simulink model "AsteroidImpact_2018a_original"  (R2019a)
settings: Solver=ode4  StartTime=0.0  StopTime=45  FixedStep=0.001  RelTol=1e-3
undefined symbols (not defined in the file or in its folder): g_, K, m_
libraries: eeGeneralControl x2
settings Model: Creator=KNMALE002  LastModifiedBy=Jamie Aronson
settings DataIOCC: SaveOutput=off  SignalLogging=off  DSMLogging=off  ReturnWorkspaceOutputs=off  TimeSaveName=simulation_time
settings DebuggingCC: ArithmeticOperatorsInVariantConditions=warning

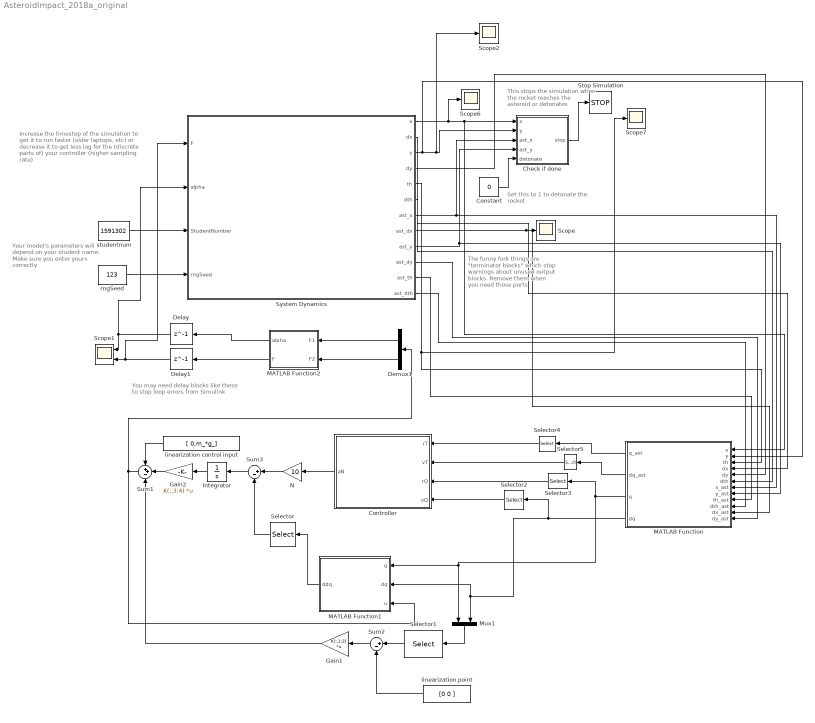
== system AsteroidImpact_2018a_original ==
  note: Increase the timestep of the simulation to get it to run faster (older laptops, etc) or decrease it to get less lag for the (discrete parts of) your controller (higher sampling rate)
  note: You may need delay blocks like these to stop loop errors from Simulink
  note: Your model's parameters will depend on your student name. Make sure you enter yours correctly
  note: The funny fork things are "terminator blocks" which stop warnings about unused output blocks. Remove them when you need those ports
  note: This stops the simulation when the rocket reaches the asteroid or detonates
  note: Set this to 1 to detonate the rocket
  Check if done : MATLAB Function  TreatAsAtomicUnit=on
  Constant : Constant  Value=0
  Controller : MATLAB Function  TreatAsAtomicUnit=on
  Delay : Delay  DelayLength=1  InitialCondition=0
  Delay1 : Delay  DelayLength=1  InitialCondition=10000
  Demux1 : Demux  Outputs=2
  Gain1 : Gain  Gain=K(:,1:2)  Multiplication=Matrix(K*u)
  Gain2 : Gain  Gain=K(:,3:4)  Multiplication=Matrix(K*u)
  Integrator : Integrator
  MATLAB Function : MATLAB Function  TreatAsAtomicUnit=on
  MATLAB Function1 : MATLAB Function  TreatAsAtomicUnit=on
  MATLAB Function2 : MATLAB Function  TreatAsAtomicUnit=on
  Mux1 : Mux  Inputs=2
  N : Gain  Gain=10
  Scope{,2,6..7} (4 alike) : Scope
  Scope1 : Scope  NumInputPorts=2
  Selector{,2..5} (5 alike) : Selector  InputPortWidth=3  IndexOptions=Index vector (dialog)  Indices=[1 2]  OutputSizes=1
  Selector1 : Selector  InputPortWidth=6  IndexOptions=Index vector (dialog)  Indices=[3 6]  OutputSizes=1
  Stop Simulation : Stop
  Sum1 : Sum  Inputs=++-
  Sum2 : Sum  Inputs=|+-
  Sum3 : Sum  Inputs=|+-
  System Dynamics : Subsystem  TreatAsAtomicUnit=on  mask{Value=1}
      mask prompts: Value "Enter mode (1, 2 or 3)"
      mask TypeOptions Value: ScenarioVar/Value
      mask Display: image('lander.jpg');
  linearization control input : Constant  Value=[ 0,m_*g_]
  linearization point : Constant  Value=[0 0 ]
  rngSeed : Constant  Value=123
  studentnum : Constant  Value=1591302
  wires:
  studentnum/1 -> System Dynamics/3(StudentNumber)
  System Dynamics/1(x) -> Scope6/1, MATLAB Function/1(x), Check if done/1(x)
  rngSeed/1 -> System Dynamics/4(rngSeed)
  System Dynamics/3(y) -> MATLAB Function/2(y), Scope2/1, Check if done/2(y)
  System Dynamics/12(ast_dth) -> MATLAB Function/10(dth_ast)
  System Dynamics/7(ast_x) -> MATLAB Function/7(x_ast), Check if done/3(ast_x)
  System Dynamics/9(ast_y) -> MATLAB Function/8(y_ast), Check if done/4(ast_y)
  System Dynamics/8(ast_dx) -> MATLAB Function/11(dx_ast), Scope/1
  System Dynamics/11(ast_th) -> MATLAB Function/9(th_ast)
  Constant/1 -> Check if done/5(detonate)
  System Dynamics/4(dy) -> MATLAB Function/5(dy)
  System Dynamics/10(ast_dy) -> MATLAB Function/12(dy_ast)
  System Dynamics/2(dx) -> MATLAB Function/4(dx)
  System Dynamics/6(dth) -> MATLAB Function/6(dth)
  MATLAB Function/1(q_ast) -> Selector4/1
  MATLAB Function/2(dq_ast) -> Selector5/1
  MATLAB Function/3(q) -> Mux1/1, MATLAB Function1/1(q), Selector3/1
  MATLAB Function/4(dq) -> MATLAB Function1/2(dq), Mux1/2, Selector2/1
  Controller/1(aN) -> N/1
  N/1 -> Sum3/1
  linearization control input/1 -> Sum1/1
  Gain2/1 -> Sum1/2
  Mux1/1 -> Selector1/1
  linearization point/1 -> Sum2/2
  Sum2/1 -> Gain1/1
  Gain1/1 -> Sum1/3
  Selector1/1 -> Sum2/1
  Sum1/1 -> MATLAB Function1/3(u), Demux1/1
  MATLAB Function1/1(ddq) -> Selector/1
  Selector/1 -> Sum3/2
  System Dynamics/5(th) -> Scope7/1, MATLAB Function/3(th)
  Selector2/1 -> Controller/4(vQ)
  Selector3/1 -> Controller/3(rQ)
  Selector4/1 -> Controller/1(rT)
  Selector5/1 -> Controller/2(vT)
  Demux1/1 -> MATLAB Function2/1(F1)
  Demux1/2 -> MATLAB Function2/2(F2)
  MATLAB Function2/2(F) -> Delay1/1
  Delay/1 -> System Dynamics/2(alpha), Scope1/1
  Integrator/1 -> Gain2/1
  Sum3/1 -> Integrator/1
  MATLAB Function2/1(alpha) -> Delay/1
  Delay1/1 -> System Dynamics/1(F), Scope1/2
  Check if done/1(stop) -> Stop Simulation/1

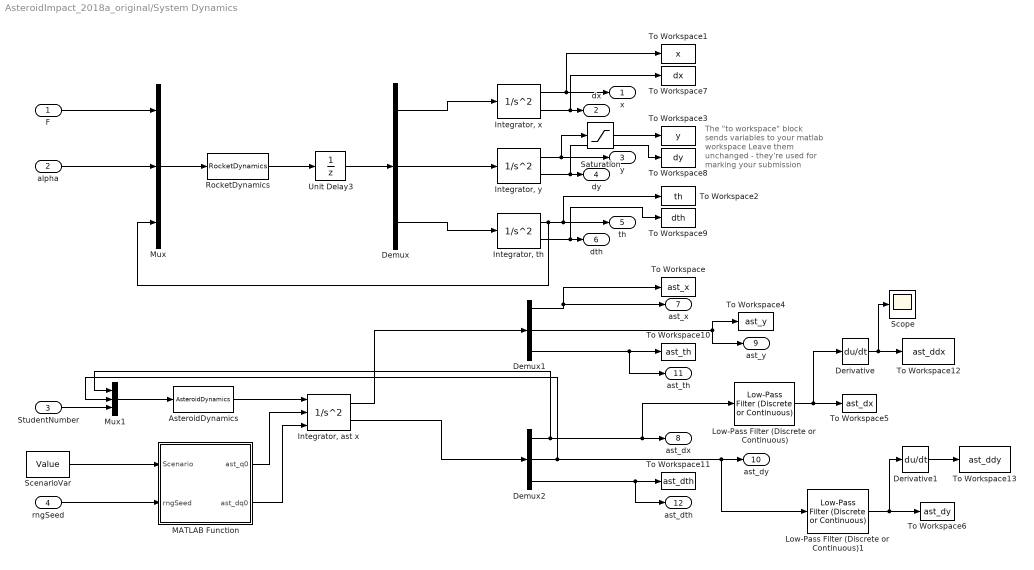
== system AsteroidImpact_2018a_original/System Dynamics ==
  note: The "to workspace" block sends variables to your matlab workspace
      |
      | Leave them unchanged - they're used for marking your submission
  F : Inport
  alpha : Inport  Port=2
  StudentNumber : Inport  Port=3
  rngSeed : Inport  Port=4
  AsteroidDynamics : MATLABFcn  MATLABFcn=AsteroidDynamics  OutputDimensions=3
  Demux : Demux  Outputs=3
  Demux1 : Demux  Outputs=3
  Demux2 : Demux  Outputs=3
  Derivative : Derivative
  Derivative1 : Derivative
  "Integrator, th" : SecondOrderIntegrator  ICX=0  ICDXDT=0
  "Integrator, x" : SecondOrderIntegrator  ICX=0
  "Integrator, y" : SecondOrderIntegrator  ICX=0
  "Integrator, ast x" : SecondOrderIntegrator  ICSourceX=external  ICX=x0  ICSourceDXDT=external
  Low-Pass Filter (Discrete or Continuous) : eeGeneralControl/Low-Pass Filter (Discrete or Continuous)  K=1  T=1  B=inf  A=-inf  Ts=0
      settings: SourceProductName=Simscape Electrical
  Low-Pass Filter (Discrete or Continuous)1 : eeGeneralControl/Low-Pass Filter (Discrete or Continuous)  K=1  T=1  B=inf  A=-inf  Ts=0
      settings: SourceProductName=Simscape Electrical
  MATLAB Function : MATLAB Function  TreatAsAtomicUnit=on
  Mux : Mux  Inputs=3
  Mux1 : Mux  Inputs=3
  RocketDynamics : MATLABFcn  MATLABFcn=RocketDynamics  Output1D=off
  Saturation : Saturate  UpperLimit=10000  LowerLimit=0
  ScenarioVar : Constant  Value=Value
  Scope : Scope
  To Workspace : ToWorkspace  VariableName=ast_x  SampleTime=-1
  To Workspace1 : ToWorkspace  VariableName=x  SampleTime=-1
  To Workspace10 : ToWorkspace  VariableName=ast_th  SampleTime=-1
  To Workspace11 : ToWorkspace  VariableName=ast_dth  SampleTime=-1
  To Workspace12 : ToWorkspace  VariableName=ast_ddx  SaveFormat=Timeseries  SampleTime=-1
  To Workspace13 : ToWorkspace  VariableName=ast_ddy  SaveFormat=Timeseries  SampleTime=-1
  To Workspace2 : ToWorkspace  VariableName=th  SampleTime=-1
  To Workspace3 : ToWorkspace  VariableName=y  SampleTime=-1
  To Workspace4 : ToWorkspace  VariableName=ast_y  SampleTime=-1
  To Workspace5 : ToWorkspace  VariableName=ast_dx  SampleTime=-1
  To Workspace6 : ToWorkspace  VariableName=ast_dy  SampleTime=-1
  To Workspace7 : ToWorkspace  VariableName=dx  SampleTime=-1
  To Workspace8 : ToWorkspace  VariableName=dy  SampleTime=-1
  To Workspace9 : ToWorkspace  VariableName=dth  SampleTime=-1
  Unit Delay3 : UnitDelay  SampleTime=-1  HasFrameUpgradeWarning=on
  x : Outport  PortDimensions=1
  dx : Outport  Port=2  PortDimensions=1
  y : Outport  Port=3  PortDimensions=1
  dy : Outport  Port=4  PortDimensions=1
  th : Outport  Port=5  PortDimensions=1
  dth : Outport  Port=6  PortDimensions=1
  ast_x : Outport  Port=7  PortDimensions=1
  ast_dx : Outport  Port=8  PortDimensions=1
  ast_y : Outport  Port=9  PortDimensions=1
  ast_dy : Outport  Port=10  PortDimensions=1
  ast_th : Outport  Port=11  PortDimensions=1
  ast_dth : Outport  Port=12  PortDimensions=1
  wires:
  "Integrator, th"/1 -> th/1, To Workspace2/1, Mux/3
  Demux/1 -> "Integrator, x"/1
  Demux/2 -> "Integrator, y"/1
  Demux/3 -> "Integrator, th"/1
  "Integrator, x"/1 -> x/1, To Workspace1/1
  "Integrator, x"/2 -> To Workspace7/1, dx/1
  "Integrator, y"/2 -> To Workspace8/1, dy/1
  "Integrator, th"/2 -> To Workspace9/1, dth/1
  Mux/1 -> RocketDynamics/1
  RocketDynamics/1 -> Unit Delay3/1
  rngSeed/1 -> MATLAB Function/2(rngSeed)
  ScenarioVar/1 -> MATLAB Function/1(Scenario)
  F/1 -> Mux/1
  alpha/1 -> Mux/2
  Demux1/3 -> To Workspace10/1, ast_th/1
  Demux2/3 -> ast_dth/1, To Workspace11/1
  Mux1/1 -> AsteroidDynamics/1
  AsteroidDynamics/1 -> "Integrator, ast x"/1
  "Integrator, ast x"/1 -> Demux1/1
  "Integrator, ast x"/2 -> Demux2/1
  Demux1/1 -> To Workspace/1, ast_x/1
  Demux2/1 -> Mux1/1, Low-Pass Filter (Discrete or Continuous)/1, ast_dx/1
  Demux2/2 -> Mux1/2, Low-Pass Filter (Discrete or Continuous)1/1, ast_dy/1
  MATLAB Function/1(ast_q0) -> "Integrator, ast x"/2
  MATLAB Function/2(ast_dq0) -> "Integrator, ast x"/3
  StudentNumber/1 -> Mux1/3
  Unit Delay3/1 -> Demux/1
  "Integrator, y"/1 -> y/1, Saturation/1
  Demux1/2 -> To Workspace4/1, ast_y/1
  Saturation/1 -> To Workspace3/1
  Low-Pass Filter (Discrete or Continuous)/1 -> Derivative/1, To Workspace5/1
  Derivative/1 -> Scope/1, To Workspace12/1
  Low-Pass Filter (Discrete or Continuous)1/1 -> Derivative1/1, To Workspace6/1
  Derivative1/1 -> To Workspace13/1

== matlab function AsteroidImpact_2018a_original/System Dynamics/MATLAB Function ==
  data: ast_q0 output; ast_dq0 output; Scenario input; rngSeed input
function [ast_q0, ast_dq0] = fcn(Scenario, rngSeed)
rng(rngSeed);
if (Scenario == 1)
    x0 = -3000;
    y0 =  5000;
    th0 =   0;
    dx0 = 182;
    dy0 = 0;
    dth0 = 0;

elseif (Scenario == 2)
    x0 = -2000 + rand_within_plus_minus(100);
    y0 = 4000 + rand_within_plus_minus(100); 
    th0 = 0;
    dx0 = 170;
    dy0 = 0;
    dth0 = 0.1;


elseif (Scenario == 3)
    x0 = -2500;
    y0 = 3000;
    th0 = 0;
    dx0 = 160;
    dy0 = 100;
    dth0 = deg2rad(rand_within_plus_minus(20)); % rad/sec

else
    error('You entered an invalid mode -- make sure Scenario = 1, 2 or 3')
end

ast_q0  = [ x0;  y0;  th0];
ast_dq0 = [dx0; dy0; dth0];

end

% calling rand_within_plus_minus(100) returns a number between -100 and 100
function n = rand_within_plus_minus(interval)
    n = (rand - 0.5) * 2 * interval;
end

== matlab function AsteroidImpact_2018a_original/Controller ==
  data: aN output; rT input; vT input; rQ input; vQ input
function aN = pNav(rT, vT, rQ, vQ)
% this produces an acceleration which the controller should track
R = rT - rQ;
Rtemp = [R; 0];
Vr = vT - vQ;
Vtemp = [Vr; 0];
omega = cross(Rtemp, Vtemp) / dot(Rtemp, Rtemp);
temp = cross(Vtemp, omega);
aN = temp(1:2);

== matlab function AsteroidImpact_2018a_original/MATLAB Function ==
  data: x input; q_ast output; y input; th input; dx input; dy input; dth input; x_ast input; y_ast input; th_ast input; dth_ast input; dx_ast input; dy_ast input; dq_ast output; q output; dq output
function [q_ast, dq_ast, q, dq] = fcn(x,y,th,dx,dy,dth,x_ast, y_ast,th_ast,dth_ast, dx_ast, dy_ast)

q_ast = [x_ast; y_ast;th_ast];
dq_ast = [dx_ast; dy_ast;dth_ast]
q = [x;y;th];
dq = [dx;dy;dth];

== matlab function AsteroidImpact_2018a_original/Check if done ==
  data: x input; stop output; y input; ast_x input; ast_y input; detonate input
function stop = fcn(x, y, ast_x, ast_y, detonate)
    % given the signal to detonate
    if detonate == 1
        stop = 1;

    % rocket has hit the asteroid
    elseif norm([x; y] - [ast_x; ast_y]) < 100
        stop = 1;
    
    % rocket has hit the ground OR asteroid is close to they city
    elseif y < 0 || ast_y < 200
        stop = 1;
    
    else
        stop = 0;
    end
end

== matlab function AsteroidImpact_2018a_original/MATLAB Function1 ==
  data: q input; dq input; u input; ddq output
function ddq = fcn(q, dq, u)
m =  1000;
g = 9.81;
I =(1/12)*m*(15^2 + 5^2)+m*4^2;

F1 = u(1);
F2 = u(2);

x = q(1);
y = q(2);
th = q(3);

dx = dq(1);
dy = dq(2);
dth = dq(3);

ddq = [(F1*cos(th)-F2*sin(th))/m;(100*F2*cos(th)-981*m+100*F1*sin(th))/(100*m);7*F1/(2*I)];

== matlab function AsteroidImpact_2018a_original/MATLAB Function2 ==
  data: alpha output; F1 input; F output; F2 input
function [alpha,F]= fcn(F1, F2)
alpha = atan(-F1/F2);
F = sqrt(F1^2 + F2^2);
